simulink model "PI"  (R2018a)
settings: Solver=VariableStepAuto  StartTime=0.0  StopTime=300  RelTol=1e-3
undefined symbols (not defined in the file): Kp, T, Ti
libraries: simulink x1
settings Model: Creator=User  LastModifiedBy=User

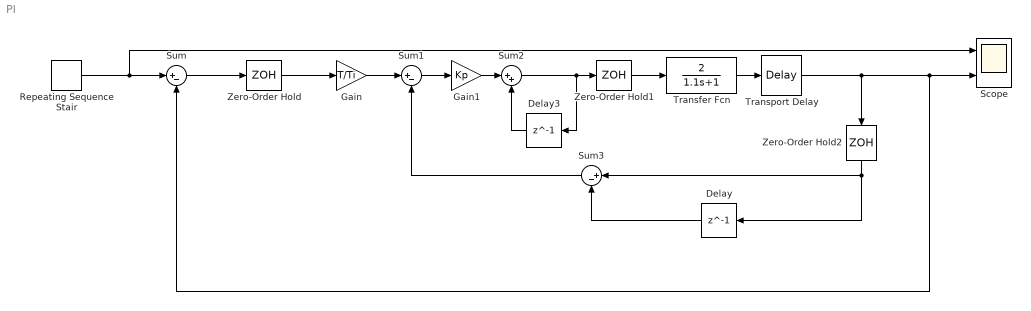
== system PI ==
  Delay : Delay  DelayLength=1
  Delay3 : Delay  DelayLength=1
  Gain : Gain  Gain=T/Ti
  Gain1 : Gain  Gain=Kp
  Repeating Sequence Stair : simulink/Sources/Repeating Sequence Stair  OutValues=[3 1 -5 2 1].'  tsamp=50  OutMin=[]  OutMax=[]  OutDataTypeStr=double  OutputDataTypeScalingMode=double  OutDataType=fixdt(0,8)  ConRadixGroup=Best Precision: Vector-wise  OutScaling=2^-12
  Scope : Scope  NumInputPorts=2
  Sum : Sum  Inputs=|+-
  Sum1 : Sum  Inputs=|+-
  Sum2 : Sum  Inputs=|++
  Sum3 : Sum  Inputs=|+-
  Transfer Fcn : TransferFcn  Numerator=[2]  Denominator=[1.1 1]
  Transport Delay : TransportDelay  DelayTime=0.773
  Zero-Order Hold : ZeroOrderHold  SampleTime=0.01
  Zero-Order Hold1 : ZeroOrderHold  SampleTime=0.01
  Zero-Order Hold2 : ZeroOrderHold  SampleTime=0.01
  wires:
  Transfer Fcn/1 -> Transport Delay/1
  Repeating Sequence Stair/1 -> Scope/1, Sum/1
  Delay/1 -> Sum3/2
  Zero-Order Hold/1 -> Gain/1
  Zero-Order Hold1/1 -> Transfer Fcn/1
  Delay3/1 -> Sum2/2
  Sum2/1 -> Delay3/1, Zero-Order Hold1/1
  Zero-Order Hold2/1 -> Delay/1, Sum3/1
  Sum3/1 -> Sum1/2
  Gain1/1 -> Sum2/1
  Sum/1 -> Zero-Order Hold/1
  Gain/1 -> Sum1/1
  Sum1/1 -> Gain1/1
  Transport Delay/1 -> Sum/2, Scope/2, Zero-Order Hold2/1
